simulink model "cnlib"  (Simulink 6.2)
settings: Solver=ode5  SolverMode=SingleTasking  StartTime=0.0  StopTime=5  FixedStep=0.001  MaxStep=0.001  RelTol=1e-3  AbsTol=1e-3
undefined symbols (not defined in the file): k
(part 3 of 7)

== system cnlib/CN SP+Sacc +BS (5/4)/IM SP + Sacc (pos-vel)/Limiter ==
  note: This block limits outputs to less than or equal to the "Limit" constant.
      | Inputs greater than "Limit" yield a zero output.
  in_1 : Inport  Port=1  LatchInput=off
  Limit : Constant  Orientation=up  Value=100
  Product : Product  SaturateOnIntegerOverflow=on  RndMeth=Zero  InputSameDT=on
  Relational Operator : RelationalOperator  Operator=<=  InputSameDT=on
  out_1 : Outport  InitialOutput=0
  wires:
  in_1/1 -> Relational Operator/1, Product/1
  Product/1 -> out_1/1
  Limit/1 -> Relational Operator/2
  Relational Operator/1 -> Product/2

== system cnlib/CN SP+Sacc +BS (5/4)/IM SP + Sacc (pos-vel)/OMN2 ==
  note: OMN
  note: Note that the OMN properly combines the pulse with the output of the NI, by latching
      | that output to its value at the moment the pulse appears.
  note: Operation: when the pulse is active ("from PG") it activates the switch, passing the
      | upper input through to the output.  When the pulse is over, the switch changes,
      | allowing the lower input (from the NI) to pass.
  note: This block behaves like the ocular motor neurons,combining a phasic pulse (from PG)
      | with the tonic step produced by integration of the step, yielding a Pulse-Step
      | to drive the plant.
  from NI : Inport  Port=1  LatchInput=off
  from PG : Inport  Port=2  LatchInput=off
  Abs : Abs  SaturateOnIntegerOverflow=on
  Gain _ : Gain  Gain=1.0  SaturateOnIntegerOverflow=on
  SampHold? : Subsystem
      mask Display: disp('S&H\n(L)')
  Sign : Subsystem
      mask Type: Sign
      mask Description: y = sign(x)
      mask Help: Sign Function:\n\t\t\ty = 1 if x > 0\n\t\t\ty = 0 if x = 0\n\t\t\ty = -1 if x < 0
      mask Display: plot(-50,-50,50,50,[-50,50],[0,0],[0,0],[-50,50],[-40,0],[-30,-30],[0,40],[30,30])
  Sum : Sum  SaturateOnIntegerOverflow=on  InputSameDT=on
  Switch : Switch  Threshold=.5  SaturateOnIntegerOverflow=on  InputSameDT=on
  out_1 : Outport  InitialOutput=0
  wires:
  from NI/1 -> Switch/3, SampHold?/1(Input)
  Sign/1(out_1) -> Switch/2, SampHold?/2(S/H?)
  Gain _/1 -> Sum/1
  SampHold?/1(output) -> Sum/2
  Sum/1 -> Switch/1
  from PG/1 -> Abs/1, Gain _/1
  Switch/1 -> out_1/1
  Abs/1 -> Sign/1(in_1)

== system cnlib/CN SP+Sacc +BS (5/4)/IM SP + Sacc (pos-vel)/Ret FB sample ==
  note: (FF init state: Q=0)
  note: * Leading Edge of a saccade DISABLEs Retinal FB
  note: Operation:
  note: * Retinal Feedback Sampling is initially ENABLED
  note: * Output of TIMER circuit REENABLES Retinal FB
  note: Retinal Feedback Sample
  _From PG : Inport  Port=1  LatchInput=off
  Latch1 : Subsystem  mask(Latch){@1=0}
      mask prompts: @1 "Initial State for Output "Q":"
      mask help: Latch
      mask init:
      | ini=(@1~=0);
      mask Help: Latches the S input.  When S (set) is one, the Q output  becomes one.  The output remains one until the R (reset) input becomes one, forcing the output to zero.  If both R and S are one, the latch will be in an undefined state.
      mask Display: disp('S   Q\n\nR  !Q')
  event timer2 : Subsystem
      mask Display: disp('Event\nTimer2')
  leading edge detect : Subsystem
      mask Display: disp('Leading\nEdge Det')
  timer value : Constant  Orientation=up  Value=.2
  out_1 : Outport  InitialOutput=0
  wires:
  timer value/1 -> event timer2/2(_timer value (port))
  _From PG/1 -> event timer2/1(_PG), leading edge detect/1(in_1)
  Latch1/2(out_2) -> out_1/1
  leading edge detect/1(out_1) -> Latch1/1(in_1)
  event timer2/1(out_1) -> Latch1/2(in_2)

== system cnlib/CN SP+Sacc +BS (5/4)/IM SP + Sacc (pos-vel)/Sacc Blank ==
  note: * Output of TIMER circuit REENABLES output
      | ("timer value" ms after end of PG)
  note: * Output is initially ENABLED
  note: Operation:
  note: Saccade Blanking
  note: (FF init state: Q=1)
  note: * Leading Edge of a saccade DISABLEs output
  _From PG : Inport  Port=1  LatchInput=off
  Latch1 : Subsystem  mask(Latch){@1=1}
      mask prompts: @1 "Initial State for Output "Q":"
      mask help: Latch
      mask init:
      | ini=(@1~=0);
      mask Help: Latches the S input.  When S (set) is one, the Q output  becomes one.  The output remains one until the R (reset) input becomes one, forcing the output to zero.  If both R and S are one, the latch will be in an undefined state.
      mask Display: disp('S   Q\n\nR  !Q')
  event timer1 : Subsystem
      mask Display: disp('Event\nTimer2')
  leading edge detect : Subsystem
      mask Display: disp('Leading\nEdge Det')
  timer value : Constant  Orientation=up  Value=.03
  out_1 : Outport  InitialOutput=0
  wires:
  leading edge detect/1(out_1) -> Latch1/2(in_2)
  event timer1/1(out_1) -> Latch1/1(in_1)
  _From PG/1 -> leading edge detect/1(in_1), event timer1/1(_PG)
  Latch1/1(out_1) -> out_1/1
  timer value/1 -> event timer1/2(_timer value (port))

== system cnlib/CN SP+Sacc +BS (5/4)/IM SP + Sacc (pos-vel)/SampHold? ==
  note: When "S/H?" is HIGH, then "Input" is switched directly to the
      | output ("sample").  When "S/H?" is LOW, the current output is
      | maintained ("hold").
  Input : Inport  Port=1  LatchInput=off
  S/H? : Inport  Port=2  LatchInput=off
  Memory : Memory  Orientation=left
  Sign : Subsystem
      mask Type: Sign
      mask Description: y = sign(x)
      mask Help: Sign Function:\n\t\t\ty = 1 if x > 0\n\t\t\ty = 0 if x = 0\n\t\t\ty = -1 if x < 0
      mask Display: plot(-50,-50,50,50,[-50,50],[0,0],[0,0],[-50,50],[-40,0],[-30,-30],[0,40],[30,30])
  Switch2 : Switch  Threshold=0.5  SaturateOnIntegerOverflow=on  InputSameDT=on
  output : Outport  InitialOutput=0
  wires:
  S/H?/1 -> Sign/1(in_1)
  Sign/1(out_1) -> Switch2/2
  Input/1 -> Switch2/1
  Switch2/1 -> output/1, Memory/1
  Memory/1 -> Switch2/3

== system cnlib/CN SP+Sacc +BS (5/4)/IM SP + Sacc (pos-vel)/SampHold?1 ==
  note: When "S/H?" is HIGH, then "Input" is switched directly to the
      | output ("sample").  When "S/H?" is LOW, the current output is
      | maintained ("hold").
  Input : Inport  Port=1  LatchInput=off
  S/H? : Inport  Port=2  LatchInput=off
  Memory : Memory  Orientation=left
  Sign : Subsystem
      mask Type: Sign
      mask Description: y = sign(x)
      mask Help: Sign Function:\n\t\t\ty = 1 if x > 0\n\t\t\ty = 0 if x = 0\n\t\t\ty = -1 if x < 0
      mask Display: plot(-50,-50,50,50,[-50,50],[0,0],[0,0],[-50,50],[-40,0],[-30,-30],[0,40],[30,30])
  Switch2 : Switch  Threshold=0.5  SaturateOnIntegerOverflow=on  InputSameDT=on
  output : Outport  InitialOutput=0
  wires:
  Memory/1 -> Switch2/3
  Input/1 -> Switch2/1
  Switch2/1 -> Memory/1, output/1
  Sign/1(out_1) -> Switch2/2
  S/H?/1 -> Sign/1(in_1)

== system cnlib/CN SP+Sacc +BS (5/4)/OMN2/SampHold? ==
  note: When "S/H?" is LOW, then "Input" is switched directly to the
      | output ("sample").  When "S/H?" is HIGH, the current output is
      | maintained ("hold").
  Input : Inport  Port=1  LatchInput=off
  S/H? : Inport  Port=2  LatchInput=off
  Memory : Memory  Orientation=left
  Sign : Subsystem
      mask Type: Sign
      mask Description: y = sign(x)
      mask Help: Sign Function:\n\t\t\ty = 1 if x > 0\n\t\t\ty = 0 if x = 0\n\t\t\ty = -1 if x < 0
      mask Display: plot(-50,-50,50,50,[-50,50],[0,0],[0,0],[-50,50],[-40,0],[-30,-30],[0,40],[30,30])
  Switch2 : Switch  Threshold=0.5  SaturateOnIntegerOverflow=on  InputSameDT=on
  output : Outport  InitialOutput=0
  wires:
  Switch2/1 -> Memory/1, output/1
  Sign/1(out_1) -> Switch2/2
  S/H?/1 -> Sign/1(in_1)
  Memory/1 -> Switch2/1
  Input/1 -> Switch2/3

== system cnlib/CN SP+Sacc +BS (5/4)/OMN2/Sign ==
  in_1 : Inport  Port=1  LatchInput=off
  Constant : Constant  Value=0
  Relational Operator : RelationalOperator  Operator=>  InputSameDT=on
  Relational Operator1 : RelationalOperator  Operator=<  InputSameDT=on
  Sum : Sum  Inputs=+-  SaturateOnIntegerOverflow=on  InputSameDT=on
  out_1 : Outport  InitialOutput=0
  wires:
  Sum/1 -> out_1/1
  Relational Operator/1 -> Sum/1
  Relational Operator1/1 -> Sum/2
  Constant/1 -> Relational Operator1/2, Relational Operator/2
  in_1/1 -> Relational Operator/1, Relational Operator1/1

== system cnlib/CN SP+Sacc +BS (5/4)/PG (simp) w/SH,latch/RefLatch (good) ==
  note: The "NOT" gate outputs a DISABLE signal whenever there is any
      | input, so that there can be no response.
  note: By ANDing these outputs, we get a signal that is DISABLED
      | starting with the beginning of the input pulse, and remains so until
      | rp milliseconds after the termination of the pulse.
  note: The falling edge" block's output becomes DISABLED upon
      | detection of the END of the input pulse, and remains
      | so until the refractory period of rp milliseconds has elapsed.
  note: It's a cheap trick, but it seems to work:
  in_1 : Inport  Port=1  LatchInput=off
  Abs : Abs  SaturateOnIntegerOverflow=on
  Logical Operator : Logic
  Logical Operator1 : Logic  Operator=NOT  Inputs=1
  trailing edge : Subsystem
      mask Display: disp('Refract\nLatch (te)')
  out_1 : Outport  InitialOutput=0
  wires:
  in_1/1 -> Abs/1
  Abs/1 -> Logical Operator1/1, trailing edge/1(in_1)
  trailing edge/1(out_1) -> Logical Operator/2
  Logical Operator1/1 -> Logical Operator/1
  Logical Operator/1 -> out_1/1

== system cnlib/CN SP+Sacc +BS (5/4)/PG (simp) w/SH,latch/SampHold?1 ==
  note: When "S/H?" is HIGH, then "Input" is switched directly to the
      | output ("sample").  When "S/H?" is LOW, the current output is
      | maintained ("hold").
  Input : Inport  Port=1  LatchInput=off
  S/H? : Inport  Port=2  LatchInput=off
  Memory : Memory  Orientation=left
  Sign : Subsystem
      mask Type: Sign
      mask Description: y = sign(x)
      mask Help: Sign Function:\n\t\t\ty = 1 if x > 0\n\t\t\ty = 0 if x = 0\n\t\t\ty = -1 if x < 0
      mask Display: plot(-50,-50,50,50,[-50,50],[0,0],[0,0],[-50,50],[-40,0],[-30,-30],[0,40],[30,30])
  Switch2 : Switch  Threshold=0.5  SaturateOnIntegerOverflow=on  InputSameDT=on
  output : Outport  InitialOutput=0
  wires:
  S/H?/1 -> Sign/1(in_1)
  Sign/1(out_1) -> Switch2/2
  Input/1 -> Switch2/1
  Switch2/1 -> output/1, Memory/1
  Memory/1 -> Switch2/3

== system cnlib/CN SP+Sacc +BS (5/4)/oscillating PMC/velocity noise2 ==
  Gain : Gain  Gain=[sqrt(Cov)]/[sqrt(Ts)]  SaturateOnIntegerOverflow=on
  White Noise : RandomNumber  Seed=seed
  Zero-Order Hold : ZeroOrderHold  SampleTime=Ts
  Out_1 : Outport  InitialOutput=0
  wires:
  Zero-Order Hold/1 -> Gain/1
  Gain/1 -> Out_1/1
  White Noise/1 -> Zero-Order Hold/1

== system cnlib/CN test parts/Tgt moved?/falling edge det ==
  note: It is also possible to remove the SIGNUM function
      | and the '==', and replace them with a simple
      | switch with a threshold of (say) 150 or so.
  note: falling edge detection
  in_1 : Inport  Port=1  LatchInput=off
  Abs : Abs  SaturateOnIntegerOverflow=on
  Derivative : Derivative
  Relational Operator : RelationalOperator  Operator===  InputSameDT=on
  Sign : Subsystem
      mask Type: Sign
      mask Description: y = sign(x)
      mask Help: Sign Function:\n\t\t\ty = 1 if x > 0\n\t\t\ty = 0 if x = 0\n\t\t\ty = -1 if x < 0
      mask Display: plot(-50,-50,50,50,[-50,50],[0,0],[0,0],[-50,50],[-40,0],[-30,-30],[0,40],[30,30])
  Threshold 1 : Constant  Value=-1
  out_1 : Outport  InitialOutput=0
  wires:
  Abs/1 -> Derivative/1
  Derivative/1 -> Sign/1(in_1)
  Sign/1(out_1) -> Relational Operator/1
  Threshold 1/1 -> Relational Operator/2
  Relational Operator/1 -> out_1/1
  in_1/1 -> Abs/1

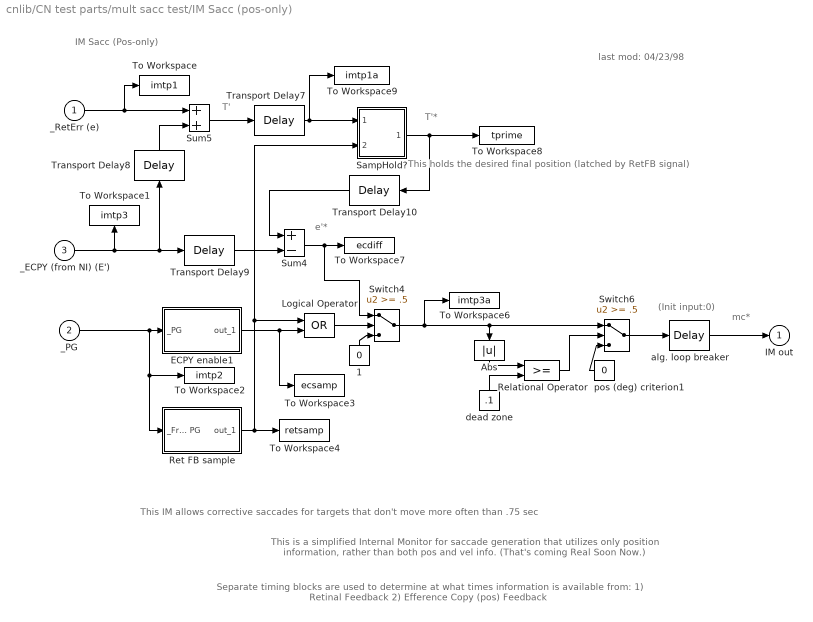
== system cnlib/CN test parts/mult sacc test/IM Sacc (pos-only) ==
  note: IM Sacc (Pos-only)
  note: This is a simplified Internal Monitor for saccade generation that utilizes only position information, rather than both pos and vel info.
      | (That's coming Real Soon Now.)
  note: Separate timing blocks are used to determine at what times information is available from:
      | 1) Retinal Feedback
      | 2) Efference Copy (pos) Feedback
  note: This IM allows corrective saccades for targets that don't move more often than .75 sec
  note: last mod:
      | 04/23/98
  note: (Init input:0)
  note: mc*
  note: T'*
  note: T'
  note: e'*
  note: This holds the desired final position
      | (latched by RetFB signal)
  _RetErr (e) : Inport  Port=1  LatchInput=off
  _PG : Inport  Port=2  LatchInput=off
  _ECPY (from NI) (E') : Inport  Port=3  LatchInput=off
  1 : Constant  Orientation=up  Value=0
  Abs : Abs  Orientation=down  SaturateOnIntegerOverflow=on
  ECPY enable1 : Subsystem
      mask Display: disp('ECPY\nEnable')
  Logical Operator : Logic  Operator=OR
  Relational Operator : RelationalOperator  InputSameDT=on
  Ret FB sample : Subsystem
      mask Display: disp('Ret FB\nEnable')
  SampHold? : Subsystem
      mask Display: disp('S&H\n(S=H)\n(H=L)')
  Sum4 : Sum  Inputs=+-  SaturateOnIntegerOverflow=on  InputSameDT=on
  Sum5 : Sum  SaturateOnIntegerOverflow=on  InputSameDT=on
  Switch4 : Switch  Threshold=.5  SaturateOnIntegerOverflow=on  InputSameDT=on
  Switch6 : Switch  Threshold=.5  SaturateOnIntegerOverflow=on  InputSameDT=on
  To Workspace : ToWorkspace  VariableName=imtp1  SaveFormat=Array
      settings: MaxDataPoints=10000
  To Workspace1 : ToWorkspace  VariableName=imtp3  SaveFormat=Array
      settings: Orientation=up  MaxDataPoints=10000
  To Workspace2 : ToWorkspace  VariableName=imtp2  SaveFormat=Array
      settings: MaxDataPoints=10000
  To Workspace3 : ToWorkspace  VariableName=ecsamp  SaveFormat=Array
      settings: MaxDataPoints=10000
      mask Type: imsw1in
  To Workspace4 : ToWorkspace  VariableName=retsamp  SaveFormat=Array
      settings: MaxDataPoints=10000
      mask Type: imsw1in
  To Workspace6 : ToWorkspace  VariableName=imtp3a  SaveFormat=Array
      settings: MaxDataPoints=10000
  To Workspace7 : ToWorkspace  VariableName=ecdiff  SaveFormat=Array
      settings: MaxDataPoints=10000
  To Workspace8 : ToWorkspace  VariableName=tprime  SaveFormat=Array
      settings: MaxDataPoints=10000
  To Workspace9 : ToWorkspace  VariableName=imtp1a  SaveFormat=Array
      settings: MaxDataPoints=10000
  Transport Delay10 : TransportDelay  Orientation=left  DelayTime=.050
      mask Display: disp('50ms')
  Transport Delay7 : TransportDelay  DelayTime=.050
      mask Display: disp('50ms')
  Transport Delay8 : TransportDelay  Orientation=up  DelayTime=0.080
      mask Display: disp('80ms')
  Transport Delay9 : TransportDelay  DelayTime=.13
      mask Display: disp('130ms')
  alg. loop breaker : TransportDelay  DelayTime=0.001
  dead zone : Constant  Orientation=up  Value=.1
  pos (deg) criterion1 : Constant  Orientation=left  Value=0
  IM out : Outport  InitialOutput=0
  wires:
  1/1 -> Switch4/3
  _PG/1 -> ECPY enable1/1(_PG), Ret FB sample/1(_From PG), To Workspace2/1
  Relational Operator/1 -> Switch6/2
  dead zone/1 -> Relational Operator/2
  pos (deg) criterion1/1 -> Switch6/3
  Abs/1 -> Relational Operator/1
  Switch6/1 -> alg. loop breaker/1
  alg. loop breaker/1 -> IM out/1
  Ret FB sample/1(out_1) -> To Workspace4/1, SampHold?/2(S/H?), Logical Operator/1
  Sum5/1 -> Transport Delay7/1
  Transport Delay9/1 -> Sum4/2
  Transport Delay8/1 -> Sum5/2
  Sum4/1 -> To Workspace7/1, Switch4/1
  _RetErr (e)/1 -> Sum5/1, To Workspace/1
  _ECPY (from NI) (E')/1 -> Transport Delay9/1, Transport Delay8/1, To Workspace1/1
  Transport Delay7/1 -> SampHold?/1(Input), To Workspace9/1
  Transport Delay10/1 -> Sum4/1
  SampHold?/1(output) -> To Workspace8/1, Transport Delay10/1
  Switch4/1 -> Switch6/1, Abs/1, To Workspace6/1
  Logical Operator/1 -> Switch4/2
  ECPY enable1/1(out_1) -> To Workspace3/1, Logical Operator/2

== system cnlib/CN test parts/mult sacc test/OMN ==
  note: Note that the OMN properly combines the pulse with the output of the NI, by latching
      | that output to its value at the moment the pulse appears.
  note: OMN
  note: Operation: when the pulse is active ("from PG") it activates the switch, passing the
      | upper input through to the output.  When the pulse is over, the switch changes,
      | allowing the lower input (from the NI) to pass.
  note: This block behaves like the ocular motor neurons,combining a phasic pulse (from PG)
      | with the tonic step produced by integration of the step, yielding a Pulse-Step
      | to drive the plant.
  from PG : Inport  Port=1  LatchInput=off
  from NI : Inport  Port=2  LatchInput=off
  Abs : Abs  SaturateOnIntegerOverflow=on
  Gain _ : Gain  Gain=1.0  SaturateOnIntegerOverflow=on
  SampHold? : Subsystem
      mask Display: disp('S&H\n(L)')
  Sign : Subsystem
      mask Type: Sign
      mask Description: y = sign(x)
      mask Help: Sign Function:\n\t\t\ty = 1 if x > 0\n\t\t\ty = 0 if x = 0\n\t\t\ty = -1 if x < 0
      mask Display: plot(-50,-50,50,50,[-50,50],[0,0],[0,0],[-50,50],[-40,0],[-30,-30],[0,40],[30,30])
  Sum : Sum  SaturateOnIntegerOverflow=on  InputSameDT=on
  Switch : Switch  Threshold=.5  SaturateOnIntegerOverflow=on  InputSameDT=on
  To Workspace : ToWorkspace  VariableName=ni_in  SaveFormat=Array
      settings: MaxDataPoints=10000
  To Workspace1 : ToWorkspace  VariableName=pg_in  SaveFormat=Array
      settings: MaxDataPoints=10000
  out_1 : Outport  InitialOutput=0
  wires:
  SampHold?/1(output) -> Sum/2
  Sign/1(out_1) -> Switch/2, SampHold?/2(S/H?)
  from PG/1 -> Abs/1, Gain _/1
  Sum/1 -> Switch/1, To Workspace1/1
  from NI/1 -> Switch/3, To Workspace/1, SampHold?/1(Input)
  Gain _/1 -> Sum/1
  Switch/1 -> out_1/1
  Abs/1 -> Sign/1(in_1)

== system cnlib/CN test parts/mult sacc test/PG (simp) w/SH,latch ==
  note: (Init input:0)
  note: (Init input:1)
  note: PG (simp) w/SH, Latch
  note: This is a somewhat simplified Pulse Generator.  It does not use feedback, as does the
      | original version, but rather uses the calculated PW and PH functions to deliver
      | a timed pulse of the specified magnitude.
  note: It is also capable of generating saccades to the left or the right, and has a piece-wise
      | linear relationship for pulse width (for saccades >1 deg and those <1 degree).
  note: While perhaps not physiological, it has the virtue of actually working
      | 1) predictably and 2) correctly, making it useful for testing of the rest of the model.
  in_1 : Inport  Port=1  LatchInput=off
  1ms (loop breaker) : TransportDelay  Orientation=left  DelayTime=0.001
  Abs : Abs  SaturateOnIntegerOverflow=on
  Constant : Constant  Value=0
  MATLAB Fcn : MATLABFcn  MATLABFcn=PWsimp
      mask Help: u>=1: y=(1.3*abs(u)+12)/1000\nu <1: y=(12*abs(u))/1000
      mask Display: disp('PW\nsimp')
  MATLAB Fcn1 : MATLABFcn  MATLABFcn=PHsimp
      mask Help: u<=0.25: y=0\nu> 0.25:  y = 590*u/(7.5+abs(u))
      mask Display: disp('PH\nsimp')
  RefLatch (good) : Subsystem  Orientation=left  mask{@1=50}
      mask prompts: @1 "Refractory Period (ms)"
      mask help: Refractory Latch
      mask init:
      | delay=@1;
      mask Display: disp('Refract\nLatch')
  SampHold?1 : Subsystem
      mask Display: disp('S&H\n(S=H)\n(H=L)')
  Sum : Sum  Inputs=+-  SaturateOnIntegerOverflow=on  InputSameDT=on
  Switch : Switch  Threshold=0.5  SaturateOnIntegerOverflow=on  InputSameDT=on
  To Workspace : ToWorkspace  VariableName=peakval  SaveFormat=Array
      settings: MaxDataPoints=10000
  To Workspace1 : ToWorkspace  VariableName=dur  SaveFormat=Array
      settings: MaxDataPoints=10000
  To Workspace2 : ToWorkspace  VariableName=pgtp1  SaveFormat=Array
      settings: MaxDataPoints=10000
  To Workspace3 : ToWorkspace  VariableName=shout  SaveFormat=Array
      settings: MaxDataPoints=10000
  To Workspace5 : ToWorkspace  VariableName=shin  SaveFormat=Array
      settings: MaxDataPoints=10000
  Variable Transport Delay : VariableTransportDelay  MaximumDelay=10  InitialInput=1
  out_1 : Outport  InitialOutput=0
  wires:
  SampHold?1/1(output) -> MATLAB Fcn1/1, MATLAB Fcn/1, To Workspace3/1
  in_1/1 -> SampHold?1/1(Input), To Workspace5/1
  MATLAB Fcn1/1 -> Switch/1, To Workspace/1, Variable Transport Delay/1, Sum/1
  Switch/1 -> 1ms (loop breaker)/1, out_1/1
  Constant/1 -> Switch/3
  Variable Transport Delay/1 -> To Workspace2/1, Sum/2
  1ms (loop breaker)/1 -> RefLatch (good)/1(in_1)
  Abs/1 -> Switch/2
  Sum/1 -> Abs/1
  MATLAB Fcn/1 -> Variable Transport Delay/2, To Workspace1/1
  RefLatch (good)/1(out_1) -> SampHold?1/2(S/H?)

== system cnlib/CN test parts/summing test/rising edge det ==
  note: rising edge detection
  note: It is also possible to remove the SIGNUM function
      | and the '==', and replace them with a simple
      | switch with a threshold of (say) 150 or so.
  in_1 : Inport  Port=1  LatchInput=off
  Abs : Abs  SaturateOnIntegerOverflow=on
  Derivative : Derivative
  Relational Operator : RelationalOperator  Operator===  InputSameDT=on
  Sign : Subsystem
      mask Type: Sign
      mask Description: y = sign(x)
      mask Help: Sign Function:\n\t\t\ty = 1 if x > 0\n\t\t\ty = 0 if x = 0\n\t\t\ty = -1 if x < 0
      mask Display: plot(-50,-50,50,50,[-50,50],[0,0],[0,0],[-50,50],[-40,0],[-30,-30],[0,40],[30,30])
  Threshold 1 : Constant
  out_1 : Outport  InitialOutput=0
  wires:
  in_1/1 -> Abs/1
  Relational Operator/1 -> out_1/1
  Threshold 1/1 -> Relational Operator/2
  Sign/1(out_1) -> Relational Operator/1
  Derivative/1 -> Sign/1(in_1)
  Abs/1 -> Derivative/1

== system cnlib/Robinson CN testing/Robinson Fig. 8'/oscillating PMC ==
  note: Robinson: PMC block
  note: motor
      | error
  note: desired
      | eye accel
  note: efference
      | copy
  note: "Acceleration saturation" can be seen as a lookup table that
      | provides an acceleration for a given input velocity.  We then
      | use an integrator to convert the acceleration back to a velocity.
  note: From: Robinson DA, Gordon JL and Gordon SE
      | A model of smooth pursuit eye movements
      | Biological Cybernetics 55: 43-57,  1986
  note: By adding a feedback gain, and
      | matching it with a feedforward gain
      | we can make this block oscillate at
      | a lower tau3 than it would otherwise.
  desired eye vel : Inport  Port=1  LatchInput=off
  Sum : Sum  Inputs=-+  SaturateOnIntegerOverflow=on  InputSameDT=on
  Transfer Fcn2 : TransferFcn  Numerator=[1.1]  Denominator=[1 0]
  accel saturation : MATLABFcn  MATLABFcn=accsat
      mask Display: plot([-80 -4 4 80],[-120 -40 40 120], [0 0],[-120 120],[-80 80],[0 0])
  feedback : Gain  Orientation=left  Gain=3.3  SaturateOnIntegerOverflow=on
  feedfwd : Gain  Gain=3.3  SaturateOnIntegerOverflow=on
  tau2 : TransportDelay  DelayTime=0.035
      mask Display: disp('35ms')
  tau3 : TransportDelay  Orientation=left  DelayTime=.025
      mask Display: disp('25ms')
  efference copy eye vel : Outport  InitialOutput=0
  wires:
  accel saturation/1 -> tau2/1
  tau2/1 -> Transfer Fcn2/1
  Sum/1 -> accel saturation/1
  tau3/1 -> Sum/1
  desired eye vel/1 -> Sum/2
  feedback/1 -> tau3/1
  feedfwd/1 -> efference copy eye vel/1
  Transfer Fcn2/1 -> feedfwd/1, feedback/1

== system cnlib/Robinson CN testing/Robinson Fig. 8'/velocity noise ==
  Gain : Gain  Gain=[sqrt(Cov)]/[sqrt(Ts)]  SaturateOnIntegerOverflow=on
  White Noise : RandomNumber  Seed=seed
  Zero-Order Hold : ZeroOrderHold  SampleTime=Ts
  Out_1 : Outport  InitialOutput=0
  wires:
  White Noise/1 -> Zero-Order Hold/1
  Gain/1 -> Out_1/1
  Zero-Order Hold/1 -> Gain/1

== system cnlib/CN IM Lib/BS Logic1/BS Enable/BS Timing ==
  note: (FF init state: Q=0)
  note: * Leading Edge of input ENABLEs output
  note: Operation:
  note: *BS Enabling is initially DISABLED
  note: * Output of TIMER circuit DISABLES output
  note: BS Timing
  From  <= [cmpr] : Inport  Port=1  LatchInput=off
  timer dur : Inport  Orientation=up  Port=2  LatchInput=off
  Latch1 : Subsystem  mask(Latch){@1=0}
      mask prompts: @1 "Initial State for Output "Q":"
      mask help: Latch
      mask init:
      | ini=(@1~=0);
      mask Help: Latches the S input.  When S (set) is one, the Q output  becomes one.  The output remains one until the R (reset) input becomes one, forcing the output to zero.  If both R and S are one, the latch will be in an undefined state.
      mask Display: disp('S   Q\n\nR  !Q')
  event timer2 : Subsystem
      mask Display: disp('Event\nTimer2')
  leading edge detect : Subsystem
      mask Display: disp('Leading\nEdge Det')
  "[bsenab]" : Outport  InitialOutput=0
  wires:
  From  <= [cmpr]/1 -> leading edge detect/1(in_1), event timer2/1(_PG)
  leading edge detect/1(out_1) -> Latch1/1(in_1)
  event timer2/1(out_1) -> Latch1/2(in_2)
  Latch1/1(out_1) -> "[bsenab]"/1
  timer dur/1 -> event timer2/2(_timer value (port))

== system cnlib/CN IM Lib/IM SP + Sacc (pos-vel)/BS Logic/BS Enable ==
  note: This block allows a BS for up to xx ms (set by "timer value")
      | after the acceleration criterion is met (i.e., drops below threshold)
  "ecdiff1 " : Inport  Port=1  LatchInput=off
  evpr : Inport  Port=2  LatchInput=off
  Abs1 : Abs  SaturateOnIntegerOverflow=on
  BS Enable : Subsystem
      mask Display: disp('BS\nEnable')
  Derivative : Derivative
      mask Display: disp('s')
  Relational Operator3 : RelationalOperator  Operator=<=  InputSameDT=on
  Switch4 : Switch  Threshold=.5  SaturateOnIntegerOverflow=on  InputSameDT=on
  To Workspace14 : ToWorkspace  VariableName=cmpr  SaveFormat=Array
      settings: MaxDataPoints=10000
      mask Type: imsw1in
  To Workspace15 : ToWorkspace  VariableName=bsenab  SaveFormat=Array
      settings: MaxDataPoints=10000
      mask Type: imsw1in
  To Workspace16 : ToWorkspace  VariableName=sout  SaveFormat=Array
      settings: MaxDataPoints=10000
      mask Type: imsw1in
  off : Constant  Orientation=up  Value=0
  threshold (accel) : Constant  Value=40
  timer value : Constant  Orientation=up  Value=.035
  ecdiff (switched) : Outport  InitialOutput=0
  wires:
  Derivative/1 -> To Workspace16/1, Abs1/1
  Abs1/1 -> Relational Operator3/1
  BS Enable/1(out_1) -> To Workspace15/1, Switch4/2
  Relational Operator3/1 -> To Workspace14/1, BS Enable/1(From >=)
  evpr/1 -> Derivative/1
  off/1 -> Switch4/3
  threshold (accel)/1 -> Relational Operator3/2
  "ecdiff1 "/1 -> Switch4/1
  Switch4/1 -> ecdiff (switched)/1
  timer value/1 -> BS Enable/2(timer dur)

== system cnlib/CN IM Lib/IM SP + Sacc (pos-vel)/BS Logic/Dead Zone [Better]1 ==
  note: This block is a better implementation of a dead zone than  the
      | block supplied by SIMULINK, because here we don't _subtract_
      | the dead zone from the rest of output.
  note: We just output zero when the dead zone is in effect, and leave the
      |  output alone the rest of the time.
  in_1 : Inport  Port=1  LatchInput=off
  Abs : Abs  Orientation=down  SaturateOnIntegerOverflow=on
  Relational Operator : RelationalOperator  InputSameDT=on
  Switch6 : Switch  Threshold=.5  SaturateOnIntegerOverflow=on  InputSameDT=on
  dead zone : Constant  Orientation=up
  pos (deg) criterion1 : Constant  Orientation=left  Value=0
  out_1 : Outport  InitialOutput=0
  wires:
  Switch6/1 -> out_1/1
  in_1/1 -> Abs/1, Switch6/1
  Abs/1 -> Relational Operator/1
  pos (deg) criterion1/1 -> Switch6/3
  dead zone/1 -> Relational Operator/2
  Relational Operator/1 -> Switch6/2

== system cnlib/CN IM Lib/IM SP + Sacc (pos-vel)/BS Logic/FS or BS? ==
  note: FS or BS?
  note: If the position error is _decreasing_, then the eye is approaching the
      | target, and we would like to generate a foveating saccade, since
      | this is our best time to consider capturing the target.
  note: The position error is compared to its value 5 milliseconds earlier.
      | If the error is _increasing_, we want to make a braking
      | saccade to oppose the runaway.
  pos error : Inport  Port=1  LatchInput=off
  Abs : Abs  SaturateOnIntegerOverflow=on
  Relational Operator : RelationalOperator  InputSameDT=on
  Transport Delay1 : TransportDelay  DelayTime=.005
      mask Display: disp('5ms')
  BS=1 FS=0 : Outport  InitialOutput=0
  wires:
  Abs/1 -> Transport Delay1/1, Relational Operator/1
  pos error/1 -> Abs/1
  Relational Operator/1 -> BS=1 FS=0/1
  Transport Delay1/1 -> Relational Operator/2

== system cnlib/CN IM Lib/IM SP + Sacc (pos-vel)/BS Logic/direction ==
  in_1 : Inport  Port=1  LatchInput=off
  Constant : Constant  Value=0
  Relational Operator : RelationalOperator  Operator=>  InputSameDT=on
  Relational Operator1 : RelationalOperator  Operator=<  InputSameDT=on
  Sum : Sum  Inputs=+-  SaturateOnIntegerOverflow=on  InputSameDT=on
  out_1 : Outport  InitialOutput=0
  wires:
  Sum/1 -> out_1/1
  Relational Operator/1 -> Sum/1
  Relational Operator1/1 -> Sum/2
  Constant/1 -> Relational Operator/2, Relational Operator1/2
  in_1/1 -> Relational Operator1/1, Relational Operator/1

== system cnlib/CN IM Lib/IM SP + Sacc (pos-vel)/ECPY enable1/ECPY sample ==
  note: This block outputs an ENABLE signal xx milliseconds long (set in "enable duration"),
      | starting xx milliseconds (set in "post-pulse delay time") AFTER the PG pulse concludes.
  note: This signal is used by the Internal Monitor to decide when to compare EFERENCE COPY
      | eye position with old eye position to decide if an appropriate saccade was made.
  note: (((see original refract latch block for full description of operation.)))
  note: (FF init state: Q=0)
  note: (Init input: 0)
  note: (FF init state: Q=0)
  note: (Init input: 1)
  note: (Init input:0)
  in_1 : Inport  Port=1  LatchInput=off
  Latch2 : Subsystem  mask(Latch){@1=0}
      mask prompts: @1 "Initial State for Output "Q":"
      mask help: Latch
      mask init:
      | ini=(@1~=0);
      mask Help: Latches the S input.  When S (set) is one, the Q output becomes one.  The output remains one until the R (reset) input becomes one, forcing the output to zero.  If both R and S are one, the latch will be in an undefined state.
      mask Display: disp('S   Q\n\nR  !Q')
  Latch4 : Subsystem  mask(Latch){@1=0}
      mask prompts: @1 "Initial State for Output "Q":"
      mask help: Latch
      mask init:
      | ini=(@1~=0);
      mask Help: Latches the S input.  When S (set) is one, the Q output becomes one.  The output remains one until the R (reset) input becomes one, forcing the output to zero.  If both R and S are one, the latch will be in an undefined state.
      mask Display: disp('S   Q\n\nR  !Q')
  Switch1 : Switch  Threshold=.5  SaturateOnIntegerOverflow=on  InputSameDT=on
  Threshold 3 : Constant  Orientation=left  Value=0
  enable duration : TransportDelay  DelayTime=.01  InitialInput=1
  leading edge detect : Subsystem
      mask Display: disp('Leading\nEdge Det')
  leading edge detect1 : Subsystem
      mask Display: disp('Leading\nEdge Det')
  loop breaker : Memory  Orientation=left
  or : Logic  Operator=OR
  post-pulse delay time : TransportDelay  DelayTime=.13
  trailing edge detect : Subsystem
      mask Display: disp('Trailing\nEdge Det')
  out_1 : Outport  InitialOutput=0
  wires:
  Latch4/1(out_1) -> leading edge detect/1(in_1)
  post-pulse delay time/1 -> Latch4/1(in_1)
  Latch2/2(out_2) -> loop breaker/1
  enable duration/1 -> Latch2/2(in_2)
  leading edge detect/1(out_1) -> enable duration/1, Latch2/1(in_1)
  Latch2/1(out_1) -> out_1/1
  loop breaker/1 -> Switch1/2
  Threshold 3/1 -> Switch1/3
  in_1/1 -> Switch1/1
  leading edge detect1/1(out_1) -> or/2
  Switch1/1 -> leading edge detect1/1(in_1), trailing edge detect/1(in_1)
  trailing edge detect/1(out_1) -> or/1, post-pulse delay time/1
  or/1 -> Latch4/2(in_2)

== system cnlib/CN IM Lib/IM SP + Sacc (pos-vel)/ECPY enable1/Latch2 ==
  in_1 : Inport  Port=1  LatchInput=off
  in_2 : Inport  Port=2  LatchInput=off
  Demux : Demux  Outputs=2
  Logic : CombinatorialLogic  TruthTable=[0 1;0 1;1 0;0 1;1 0;0 1;1 0;1 0]
  Memory : Memory  Orientation=left  X0=ini
  Mux : Mux  Inputs=3
  out_1 : Outport  InitialOutput=0
  out_2 : Outport  Port=2  InitialOutput=0
  wires:
  in_2/1 -> Mux/3
  in_1/1 -> Mux/2
  Memory/1 -> Mux/1
  Demux/1 -> Memory/1, out_1/1
  Mux/1 -> Logic/1
  Logic/1 -> Demux/1
  Demux/2 -> out_2/1

== system cnlib/CN IM Lib/IM SP + Sacc (pos-vel)/OMN2/SampHold? ==
  note: When "S/H?" is LOW, then "Input" is switched directly to the
      | output ("sample").  When "S/H?" is HIGH, the current output is
      | maintained ("hold").
  Input : Inport  Port=1  LatchInput=off
  S/H? : Inport  Port=2  LatchInput=off
  Memory : Memory  Orientation=left
  Sign : Subsystem
      mask Type: Sign
      mask Description: y = sign(x)
      mask Help: Sign Function:\n\t\t\ty = 1 if x > 0\n\t\t\ty = 0 if x = 0\n\t\t\ty = -1 if x < 0
      mask Display: plot(-50,-50,50,50,[-50,50],[0,0],[0,0],[-50,50],[-40,0],[-30,-30],[0,40],[30,30])
  Switch2 : Switch  Threshold=0.5  SaturateOnIntegerOverflow=on  InputSameDT=on
  output : Outport  InitialOutput=0
  wires:
  Input/1 -> Switch2/3
  Memory/1 -> Switch2/1
  S/H?/1 -> Sign/1(in_1)
  Sign/1(out_1) -> Switch2/2
  Switch2/1 -> output/1, Memory/1

== system cnlib/CN IM Lib/IM SP + Sacc (pos-vel)/OMN2/Sign ==
  in_1 : Inport  Port=1  LatchInput=off
  Constant : Constant  Value=0
  Relational Operator : RelationalOperator  Operator=>  InputSameDT=on
  Relational Operator1 : RelationalOperator  Operator=<  InputSameDT=on
  Sum : Sum  Inputs=+-  SaturateOnIntegerOverflow=on  InputSameDT=on
  out_1 : Outport  InitialOutput=0
  wires:
  in_1/1 -> Relational Operator1/1, Relational Operator/1
  Constant/1 -> Relational Operator/2, Relational Operator1/2
  Relational Operator1/1 -> Sum/2
  Relational Operator/1 -> Sum/1
  Sum/1 -> out_1/1

== system cnlib/CN IM Lib/IM SP + Sacc (pos-vel)/Ret FB sample/Latch1 ==
  in_1 : Inport  Port=1  LatchInput=off
  in_2 : Inport  Port=2  LatchInput=off
  Demux : Demux  Outputs=2
  Logic : CombinatorialLogic  TruthTable=[0 1;0 1;1 0;0 1;1 0;0 1;1 0;1 0]
  Memory : Memory  Orientation=left  X0=ini
  Mux : Mux  Inputs=3
  out_1 : Outport  InitialOutput=0
  out_2 : Outport  Port=2  InitialOutput=0
  wires:
  Demux/2 -> out_2/1
  Logic/1 -> Demux/1
  Mux/1 -> Logic/1
  Demux/1 -> Memory/1, out_1/1
  Memory/1 -> Mux/1
  in_1/1 -> Mux/2
  in_2/1 -> Mux/3

== system cnlib/CN IM Lib/IM SP + Sacc (pos-vel)/Ret FB sample/event timer2 ==
  note: In 2) Subsequent events DO NOT reset the counter; it only resets when it
      | reaches zero
  note: 2) A new event (leading or trailing edge) is detected. -- Only case 1)
  note: 1) The count reaches its limit (set in "timer value") -- Both case 1) and 2)
  note: In 1), Any event (leading or trailing edge) will reset the counter so that it
      | counts down from the end trailing edge) of that event.
  note: It has TWO modes: 1) Event resettable and 2) Event Non-resettable
  note: The real trick here is understanding how to reload the countdown.
      | It resets if either of two conditions is met:
  note: The "OR" gate allows either of these conditions to reset the circuit.  The delay before the
      | "S" input of the flip-flop prevents both "S" and "R" from being set simultaneously, because
      | this would put the flip-flop in an undefined state.
  note: Therefore, an event first RESETS and then SETS the flip-flop.
  note: (Init input: 0)
  note: (FF init state: Q=0)
  note: (Init input: 0)
  note: This block is an RESETTABLE EVENT TIMER.  It outputs a spike of unit height xx milliseconds
      | (set by "timer value") after it detects an event ( i.e a TRAILING edge which represents the end of a
      |  saccadic pulse)
  note: Resettable
      | Event Timer
  _PG : Inport  Port=1  LatchInput=off
  _timer value (port) : Inport  Port=2  LatchInput=off
  1 msec : TransportDelay  DelayTime=.001
  Clock : Clock
      settings: Decimation=10
  Latch1 : Subsystem  mask(Latch){@1=0}
      mask prompts: @1 "Initial State for Output "Q":"
      mask help: Latch
      mask init:
      | ini=(@1~=0);
      mask Help: Latches the S input.  When S (set) is one, the Q output  becomes one.  The output remains one until the R (reset) input becomes one, forcing the output to zero.  If both R and S are one, the latch will be in an undefined state.
      mask Display: disp('S   Q\n\nR  !Q')
  Logical Operator : Logic  Operator=OR  Inputs=3
  Logical Operator1 : Logic
  Logical Operator2 : Logic
  Relational Operator : RelationalOperator  InputSameDT=on
  SampHold?1 : Subsystem
      mask Display: disp('S&H\n(S=L)\n(H=H)')
  Sum : Sum  Inputs=+-  SaturateOnIntegerOverflow=on  InputSameDT=on
  event resettable? : Constant  Orientation=up
  leading edge detect : Subsystem
      mask Display: disp('Leading\nEdge Det')
  loop breaker : Memory  Orientation=left
  trailing edge detect : Subsystem
      mask Display: disp('Trailing\nEdge Det')
  out_1 : Outport  InitialOutput=0
  wires:
  event resettable?/1 -> Logical Operator2/2, Logical Operator1/2
  leading edge detect/1(out_1) -> Logical Operator2/1
  Logical Operator2/1 -> Logical Operator/2
  trailing edge detect/1(out_1) -> Logical Operator1/1, 1 msec/1
  Logical Operator1/1 -> Logical Operator/1
  loop breaker/1 -> Logical Operator/3
  _PG/1 -> leading edge detect/1(in_1), trailing edge detect/1(in_1)
  Latch1/1(out_1) -> SampHold?1/2(S/H?)
  Relational Operator/1 -> out_1/1, loop breaker/1
  Sum/1 -> Relational Operator/1
  Clock/1 -> Sum/1, SampHold?1/1(Input)
  SampHold?1/1(output) -> Sum/2
  Logical Operator/1 -> Latch1/2(in_2)
  1 msec/1 -> Latch1/1(in_1)
  _timer value (port)/1 -> Relational Operator/2

== system cnlib/CN IM Lib/IM SP + Sacc (pos-vel)/Ret FB sample/leading edge detect ==
  note: leading edge detection
  in_1 : Inport  Port=1  LatchInput=off
  Abs : Abs  SaturateOnIntegerOverflow=on
  Derivative : Derivative
  Relational Operator : RelationalOperator  Operator===  InputSameDT=on
  Sign : Subsystem
      mask Type: Sign
      mask Description: y = sign(x)
      mask Help: Sign Function:\n\t\t\ty = 1 if x > 0\n\t\t\ty = 0 if x = 0\n\t\t\ty = -1 if x < 0
      mask Display: plot(-50,-50,50,50,[-50,50],[0,0],[0,0],[-50,50],[-40,0],[-30,-30],[0,40],[30,30])
  Threshold 1 : Constant
  out_1 : Outport  InitialOutput=0
  wires:
  Abs/1 -> Derivative/1
  Derivative/1 -> Sign/1(in_1)
  Sign/1(out_1) -> Relational Operator/1
  Threshold 1/1 -> Relational Operator/2
  Relational Operator/1 -> out_1/1
  in_1/1 -> Abs/1

== system cnlib/CN IM Lib/IM SP + Sacc (pos-vel)/Sacc Blank/Latch1 ==
  in_1 : Inport  Port=1  LatchInput=off
  in_2 : Inport  Port=2  LatchInput=off
  Demux : Demux  Outputs=2
  Logic : CombinatorialLogic  TruthTable=[0 1;0 1;1 0;0 1;1 0;0 1;1 0;1 0]
  Memory : Memory  Orientation=left  X0=ini
  Mux : Mux  Inputs=3
  out_1 : Outport  InitialOutput=0
  out_2 : Outport  Port=2  InitialOutput=0
  wires:
  in_2/1 -> Mux/3
  in_1/1 -> Mux/2
  Memory/1 -> Mux/1
  Demux/1 -> Memory/1, out_1/1
  Mux/1 -> Logic/1
  Logic/1 -> Demux/1
  Demux/2 -> out_2/1

== system cnlib/CN IM Lib/IM SP + Sacc (pos-vel)/Sacc Blank/event timer1 ==
  note: Resettable
      | Event Timer
  note: This block is an RESETTABLE EVENT TIMER.  It outputs a spike of unit height xx milliseconds
      | (set by "timer value") after it detects an event ( i.e a TRAILING edge which represents the end of a
      |  saccadic pulse)
  note: (Init input: 0)
  note: (FF init state: Q=0)
  note: (Init input: 0)
  note: Therefore, an event first RESETS and then SETS the flip-flop.
  note: The "OR" gate allows either of these conditions to reset the circuit.  The delay before the
      | "S" input of the flip-flop prevents both "S" and "R" from being set simultaneously, because
      | this would put the flip-flop in an undefined state.
  note: The real trick here is understanding how to reload the countdown.
      | It resets if either of two conditions is met:
  note: It has TWO modes: 1) Event resettable and 2) Event Non-resettable
  note: In 1), Any event (leading or trailing edge) will reset the counter so that it
      | counts down from the end trailing edge) of that event.
  note: 1) The count reaches its limit (set in "timer value") -- Both case 1) and 2)
  note: 2) A new event (leading or trailing edge) is detected. -- Only case 1)
  note: In 2) Subsequent events DO NOT reset the counter; it only resets when it
      | reaches zero
  _PG : Inport  Port=1  LatchInput=off
  _timer value (port) : Inport  Port=2  LatchInput=off
  1 msec : TransportDelay  DelayTime=.001
  Clock : Clock
      settings: Decimation=10
  Latch1 : Subsystem  mask(Latch){@1=0}
      mask prompts: @1 "Initial State for Output "Q":"
      mask help: Latch
      mask init:
      | ini=(@1~=0);
      mask Help: Latches the S input.  When S (set) is one, the Q output  becomes one.  The output remains one until the R (reset) input becomes one, forcing the output to zero.  If both R and S are one, the latch will be in an undefined state.
      mask Display: disp('S   Q\n\nR  !Q')
  Logical Operator : Logic  Operator=OR  Inputs=3
  Logical Operator1 : Logic
  Logical Operator2 : Logic
  Relational Operator : RelationalOperator  InputSameDT=on
  SampHold?1 : Subsystem
      mask Display: disp('S&H\n(S=L)\n(H=H)')
  Sum : Sum  Inputs=+-  SaturateOnIntegerOverflow=on  InputSameDT=on
  event resettable? : Constant  Orientation=up
  leading edge detect : Subsystem
      mask Display: disp('Leading\nEdge Det')
  loop breaker : Memory  Orientation=left
  trailing edge detect : Subsystem
      mask Display: disp('Trailing\nEdge Det')
  out_1 : Outport  InitialOutput=0
  wires:
  _timer value (port)/1 -> Relational Operator/2
  1 msec/1 -> Latch1/1(in_1)
  Logical Operator/1 -> Latch1/2(in_2)
  SampHold?1/1(output) -> Sum/2
  Relational Operator/1 -> loop breaker/1, out_1/1
  _PG/1 -> trailing edge detect/1(in_1), leading edge detect/1(in_1)
  Clock/1 -> Sum/1, SampHold?1/1(Input)
  Sum/1 -> Relational Operator/1
  Latch1/1(out_1) -> SampHold?1/2(S/H?)
  loop breaker/1 -> Logical Operator/3
  Logical Operator1/1 -> Logical Operator/1
  trailing edge detect/1(out_1) -> Logical Operator1/1, 1 msec/1
  Logical Operator2/1 -> Logical Operator/2
  leading edge detect/1(out_1) -> Logical Operator2/1
  event resettable?/1 -> Logical Operator2/2, Logical Operator1/2

== system cnlib/CN IM Lib/IM SP + Sacc (pos-vel)/Sacc Blank/leading edge detect ==
  note: leading edge detection
  in_1 : Inport  Port=1  LatchInput=off
  Abs : Abs  SaturateOnIntegerOverflow=on
  Derivative : Derivative
  Relational Operator : RelationalOperator  Operator===  InputSameDT=on
  Sign : Subsystem
      mask Type: Sign
      mask Description: y = sign(x)
      mask Help: Sign Function:\n\t\t\ty = 1 if x > 0\n\t\t\ty = 0 if x = 0\n\t\t\ty = -1 if x < 0
      mask Display: plot(-50,-50,50,50,[-50,50],[0,0],[0,0],[-50,50],[-40,0],[-30,-30],[0,40],[30,30])
  Threshold 1 : Constant
  out_1 : Outport  InitialOutput=0
  wires:
  in_1/1 -> Abs/1
  Relational Operator/1 -> out_1/1
  Threshold 1/1 -> Relational Operator/2
  Sign/1(out_1) -> Relational Operator/1
  Derivative/1 -> Sign/1(in_1)
  Abs/1 -> Derivative/1

== system cnlib/CN IM Lib/IM SP + Sacc (pos-vel)/SampHold?/Sign ==
  in_1 : Inport  Port=1  LatchInput=off
  Constant : Constant  Value=0
  Relational Operator : RelationalOperator  Operator=>  InputSameDT=on
  Relational Operator1 : RelationalOperator  Operator=<  InputSameDT=on
  Sum : Sum  Inputs=+-  SaturateOnIntegerOverflow=on  InputSameDT=on
  out_1 : Outport  InitialOutput=0
  wires:
  in_1/1 -> Relational Operator1/1, Relational Operator/1
  Constant/1 -> Relational Operator/2, Relational Operator1/2
  Relational Operator1/1 -> Sum/2
  Relational Operator/1 -> Sum/1
  Sum/1 -> out_1/1

== system cnlib/CN IM Lib/IM SP + Sacc (pos-vel)/SampHold?1/Sign ==
  in_1 : Inport  Port=1  LatchInput=off
  Constant : Constant  Value=0
  Relational Operator : RelationalOperator  Operator=>  InputSameDT=on
  Relational Operator1 : RelationalOperator  Operator=<  InputSameDT=on
  Sum : Sum  Inputs=+-  SaturateOnIntegerOverflow=on  InputSameDT=on
  out_1 : Outport  InitialOutput=0
  wires:
  Sum/1 -> out_1/1
  Relational Operator/1 -> Sum/1
  Relational Operator1/1 -> Sum/2
  Constant/1 -> Relational Operator/2, Relational Operator1/2
  in_1/1 -> Relational Operator1/1, Relational Operator/1

== system cnlib/CN IM Lib/IM Sacc (pos-vel) (good!)/BS Logic/BS Enable ==
  "ecdiff1 " : Inport  Port=1  LatchInput=off
  evpr : Inport  Port=2  LatchInput=off
  Abs1 : Abs  SaturateOnIntegerOverflow=on
  BS Enable : Subsystem
      mask Display: disp('BS\nEnable')
  Derivative : Derivative
      mask Display: disp('s')
  Relational Operator3 : RelationalOperator  Operator=<=  InputSameDT=on
  Switch4 : Switch  Threshold=.5  SaturateOnIntegerOverflow=on  InputSameDT=on
  To Workspace14 : ToWorkspace  VariableName=cmpr  SaveFormat=Array
      settings: MaxDataPoints=10000
      mask Type: imsw1in
  To Workspace15 : ToWorkspace  VariableName=bsenab  SaveFormat=Array
      settings: MaxDataPoints=10000
      mask Type: imsw1in
  To Workspace16 : ToWorkspace  VariableName=sout  SaveFormat=Array
      settings: MaxDataPoints=10000
      mask Type: imsw1in
  off : Constant  Orientation=up  Value=0
  threshold (accel) : Constant  Orientation=left  Value=40
  ecdiff (switched) : Outport  InitialOutput=0
  wires:
  Derivative/1 -> Abs1/1, To Workspace16/1
  Abs1/1 -> Relational Operator3/1
  Relational Operator3/1 -> BS Enable/1(From >=), To Workspace14/1
  evpr/1 -> Derivative/1
  off/1 -> Switch4/3
  BS Enable/1(out_1) -> To Workspace15/1, Switch4/2
  threshold (accel)/1 -> Relational Operator3/2
  "ecdiff1 "/1 -> Switch4/1
  Switch4/1 -> ecdiff (switched)/1

== system cnlib/CN IM Lib/IM Sacc (pos-vel) (good!)/BS Logic/Dead Zone [Better]1 ==
  note: This block is a better implementation of a dead zone than  the
      | block supplied by SIMULINK, because here we don't _subtract_
      | the dead zone from the rest of output.
  note: We just output zero when the dead zone is in effect, and leave the
      |  output alone the rest of the time.
  in_1 : Inport  Port=1  LatchInput=off
  Abs : Abs  Orientation=down  SaturateOnIntegerOverflow=on
  Relational Operator : RelationalOperator  InputSameDT=on
  Switch6 : Switch  Threshold=.5  SaturateOnIntegerOverflow=on  InputSameDT=on
  dead zone : Constant  Orientation=up
  pos (deg) criterion1 : Constant  Orientation=left  Value=0
  out_1 : Outport  InitialOutput=0
  wires:
  Switch6/1 -> out_1/1
  in_1/1 -> Switch6/1, Abs/1
  Abs/1 -> Relational Operator/1
  pos (deg) criterion1/1 -> Switch6/3
  dead zone/1 -> Relational Operator/2
  Relational Operator/1 -> Switch6/2

== system cnlib/CN IM Lib/IM Sacc (pos-vel) (good!)/BS Logic/FS or BS? ==
  note: FS or BS?
  note: If the position error is _decreasing_, then the eye is approaching the
      | target, and we would like to generate a foveating saccade, since
      | this is our best time to consider capturing the target.
  note: The position error is compared to its value 5 milliseconds earlier.
      | If the error is _increasing_, we want to make a braking
      | saccade to oppose the runaway.
  pos error : Inport  Port=1  LatchInput=off
  Abs : Abs  SaturateOnIntegerOverflow=on
  Relational Operator : RelationalOperator  InputSameDT=on
  Transport Delay1 : TransportDelay  DelayTime=.005
      mask Display: disp('5ms')
  BS=1 FS=0 : Outport  InitialOutput=0
  wires:
  Abs/1 -> Relational Operator/1, Transport Delay1/1
  pos error/1 -> Abs/1
  Relational Operator/1 -> BS=1 FS=0/1
  Transport Delay1/1 -> Relational Operator/2

== system cnlib/CN IM Lib/IM Sacc (pos-vel) (good!)/BS Logic/direction ==
  in_1 : Inport  Port=1  LatchInput=off
  Constant : Constant  Value=0
  Relational Operator : RelationalOperator  Operator=>  InputSameDT=on
  Relational Operator1 : RelationalOperator  Operator=<  InputSameDT=on
  Sum : Sum  Inputs=+-  SaturateOnIntegerOverflow=on  InputSameDT=on
  out_1 : Outport  InitialOutput=0
  wires:
  Sum/1 -> out_1/1
  Relational Operator/1 -> Sum/1
  Relational Operator1/1 -> Sum/2
  Constant/1 -> Relational Operator1/2, Relational Operator/2
  in_1/1 -> Relational Operator/1, Relational Operator1/1

== system cnlib/CN IM Lib/IM Sacc (pos-vel) (good!)/ECPY enable1/ECPY sample ==
  note: This block outputs an ENABLE signal xx milliseconds long (set in "enable duration"),
      | starting xx milliseconds (set in "post-pulse delay time") AFTER the PG pulse concludes.
  note: This signal is used by the Internal Monitor to decide when to compare EFERENCE COPY
      | eye position with old eye position to decide if an appropriate saccade was made.
  note: (((see original refract latch block for full description of operation.)))
  note: (FF init state: Q=0)
  note: (Init input: 0)
  note: (FF init state: Q=0)
  note: (Init input: 1)
  note: (Init input:0)
  in_1 : Inport  Port=1  LatchInput=off
  Latch2 : Subsystem  mask(Latch){@1=0}
      mask prompts: @1 "Initial State for Output "Q":"
      mask help: Latch
      mask init:
      | ini=(@1~=0);
      mask Help: Latches the S input.  When S (set) is one, the Q output becomes one.  The output remains one until the R (reset) input becomes one, forcing the output to zero.  If both R and S are one, the latch will be in an undefined state.
      mask Display: disp('S   Q\n\nR  !Q')
  Latch4 : Subsystem  mask(Latch){@1=0}
      mask prompts: @1 "Initial State for Output "Q":"
      mask help: Latch
      mask init:
      | ini=(@1~=0);
      mask Help: Latches the S input.  When S (set) is one, the Q output becomes one.  The output remains one until the R (reset) input becomes one, forcing the output to zero.  If both R and S are one, the latch will be in an undefined state.
      mask Display: disp('S   Q\n\nR  !Q')
  Switch1 : Switch  Threshold=.5  SaturateOnIntegerOverflow=on  InputSameDT=on
  Threshold 3 : Constant  Orientation=left  Value=0
  enable duration : TransportDelay  DelayTime=.01  InitialInput=1
  leading edge detect : Subsystem
      mask Display: disp('Leading\nEdge Det')
  leading edge detect1 : Subsystem
      mask Display: disp('Leading\nEdge Det')
  loop breaker : Memory  Orientation=left
  or : Logic  Operator=OR
  post-pulse delay time : TransportDelay  DelayTime=.13
  trailing edge detect : Subsystem
      mask Display: disp('Trailing\nEdge Det')
  out_1 : Outport  InitialOutput=0
  wires:
  Latch4/1(out_1) -> leading edge detect/1(in_1)
  post-pulse delay time/1 -> Latch4/1(in_1)
  Latch2/2(out_2) -> loop breaker/1
  enable duration/1 -> Latch2/2(in_2)
  leading edge detect/1(out_1) -> Latch2/1(in_1), enable duration/1
  Latch2/1(out_1) -> out_1/1
  loop breaker/1 -> Switch1/2
  Threshold 3/1 -> Switch1/3
  in_1/1 -> Switch1/1
  leading edge detect1/1(out_1) -> or/2
  Switch1/1 -> trailing edge detect/1(in_1), leading edge detect1/1(in_1)
  trailing edge detect/1(out_1) -> post-pulse delay time/1, or/1
  or/1 -> Latch4/2(in_2)
